simulink model "error"  (R2020b)
settings: Solver=VariableStepAuto  StartTime=0.0  StopTime=200  RelTol=1e-3
libraries: simulink x7
settings Model: Creator=Acer  LastModifiedBy=Acer

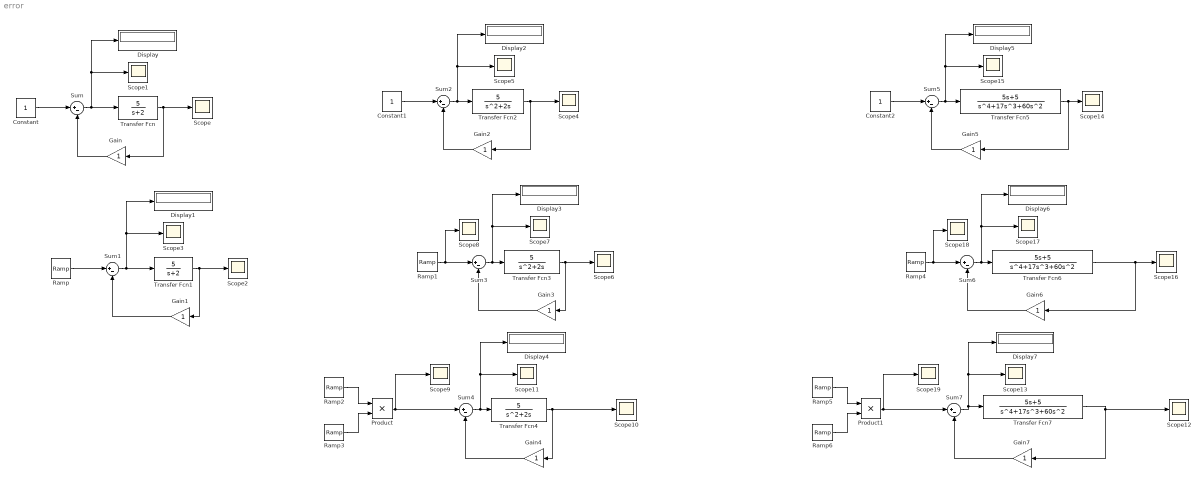
== system error ==
  Constant : Constant
  Constant1 : Constant
  Constant2 : Constant
  Display{,1..7} (8 alike) : Display
      settings: Decimation=3
  Gain{,1..7} (8 alike) : Gain
  Product : Product
  Product1 : Product
  Ramp : simulink/Sources/Ramp  slope=1  start=0  InitialOutput=0
  Ramp1 : simulink/Sources/Ramp  slope=6  start=0  InitialOutput=0
  Ramp2 : simulink/Sources/Ramp  slope=1/4  start=0  InitialOutput=0
  Ramp3 : simulink/Sources/Ramp  slope=2  start=0  InitialOutput=0
  Ramp4 : simulink/Sources/Ramp  slope=6  start=0  InitialOutput=0
  Ramp5 : simulink/Sources/Ramp  slope=1/4  start=0  InitialOutput=0
  Ramp6 : simulink/Sources/Ramp  slope=2  start=0  InitialOutput=0
  Scope{,1..19} (20 alike) : Scope
  Sum{,1..7} (8 alike) : Sum  Inputs=|+-
  Transfer Fcn : TransferFcn  Numerator=[5]  Denominator=[1 2]
  Transfer Fcn1 : TransferFcn  Numerator=[5]  Denominator=[1 2]
  Transfer Fcn2 : TransferFcn  Numerator=[5]  Denominator=[1 2 0]
  Transfer Fcn3 : TransferFcn  Numerator=[5]  Denominator=[1 2 0]
  Transfer Fcn4 : TransferFcn  Numerator=[5]  Denominator=[1 2 0]
  Transfer Fcn5 : TransferFcn  Numerator=[5 5]  Denominator=[1 17 60 0 0]
  Transfer Fcn6 : TransferFcn  Numerator=[5 5]  Denominator=[1 17 60 0 0]
  Transfer Fcn7 : TransferFcn  Numerator=[5 5]  Denominator=[1 17 60 0 0]
  wires:
  Sum/1 -> Display/1, Scope1/1, Transfer Fcn/1
  Gain/1 -> Sum/2
  Transfer Fcn/1 -> Scope/1, Gain/1
  Constant/1 -> Sum/1
  Ramp/1 -> Sum1/1
  Sum1/1 -> Display1/1, Scope3/1, Transfer Fcn1/1
  Transfer Fcn1/1 -> Scope2/1, Gain1/1
  Gain1/1 -> Sum1/2
  Ramp1/1 -> Scope8/1, Sum3/1
  Gain3/1 -> Sum3/2
  Transfer Fcn3/1 -> Scope6/1, Gain3/1
  Constant1/1 -> Sum2/1
  Sum2/1 -> Display2/1, Scope5/1, Transfer Fcn2/1
  Transfer Fcn2/1 -> Scope4/1, Gain2/1
  Gain2/1 -> Sum2/2
  Sum3/1 -> Display3/1, Scope7/1, Transfer Fcn3/1
  Ramp2/1 -> Product/1
  Ramp3/1 -> Product/2
  Product/1 -> Sum4/1, Scope9/1
  Transfer Fcn4/1 -> Scope10/1, Gain4/1
  Gain4/1 -> Sum4/2
  Sum4/1 -> Display4/1, Scope11/1, Transfer Fcn4/1
  Sum7/1 -> Transfer Fcn7/1, Display7/1, Scope13/1
  Ramp5/1 -> Product1/1
  Ramp6/1 -> Product1/2
  Gain5/1 -> Sum5/2
  Transfer Fcn7/1 -> Scope12/1, Gain7/1
  Sum5/1 -> Display5/1, Scope15/1, Transfer Fcn5/1
  Transfer Fcn5/1 -> Scope14/1, Gain5/1
  Constant2/1 -> Sum5/1
  Gain6/1 -> Sum6/2
  Ramp4/1 -> Scope18/1, Sum6/1
  Transfer Fcn6/1 -> Scope16/1, Gain6/1
  Sum6/1 -> Transfer Fcn6/1, Display6/1, Scope17/1
  Product1/1 -> Sum7/1, Scope19/1
  Gain7/1 -> Sum7/2
